simulink model "chain_CPG_2021a"  (R2021b)
settings: Solver=VariableStepAuto  StartTime=0.0  StopTime=10  RelTol=1e-3
values from neighbouring files (symbols this model uses):
  ar = 2    [Snake5animal.m]    (also in animal.m; parameters.m)
  ax = 2    [Snake5animal.m]    (also in animal.m; parameters.m)
  l = 1    [Snake5animal.m]    (also in animal.m = 0.5; parameters.m)
  N = 5    [Snake5animal.m]
  omega = ones(1,N)*0.6*pi    [Snake5animal.m]    (also in animal.m = ones(3,3)*2; parameters.m = ones(3,3)*2)
  omega1 = 0.6*pi    (= 1.88495559215)    [animal.m]    (also in parameters.m)
  omega2 = 0.6*pi    (= 1.88495559215)    [animal.m]    (also in parameters.m)
  omega3 = 0.6*pi    (= 1.88495559215)    [animal.m]    (also in parameters.m)
  phi = ones(3,3)*PHI    [animal.m]    (also in parameters.m)
  R1 = R1    [animal.m]    (also in parameters.m = 0.5708)
  R2 = R2    [animal.m]    (also in parameters.m = 0.5348)
  R3 = R3    [animal.m]    (also in parameters.m = 0.3731)
  X = zeros(1,N)    [Snake5animal.m]
  X1 = 0    [animal.m]    (also in parameters.m)
  X2 = 0    [animal.m]    (also in parameters.m)
  X3 = 0    [animal.m]    (also in parameters.m)
undefined symbols (not defined in the file or in its folder): Y, Z
libraries: sm_lib x23, nesl_utility x6
(part 1 of 2)
settings Model: Creator=xizh0002  LastModifiedBy=xizh0002

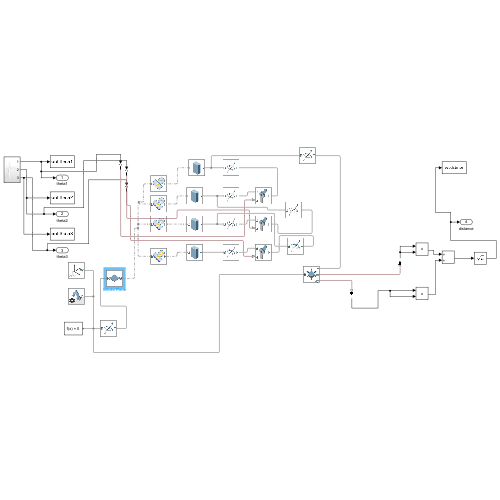
[thumbnail: Simulink's stored preview of the top-level diagram]
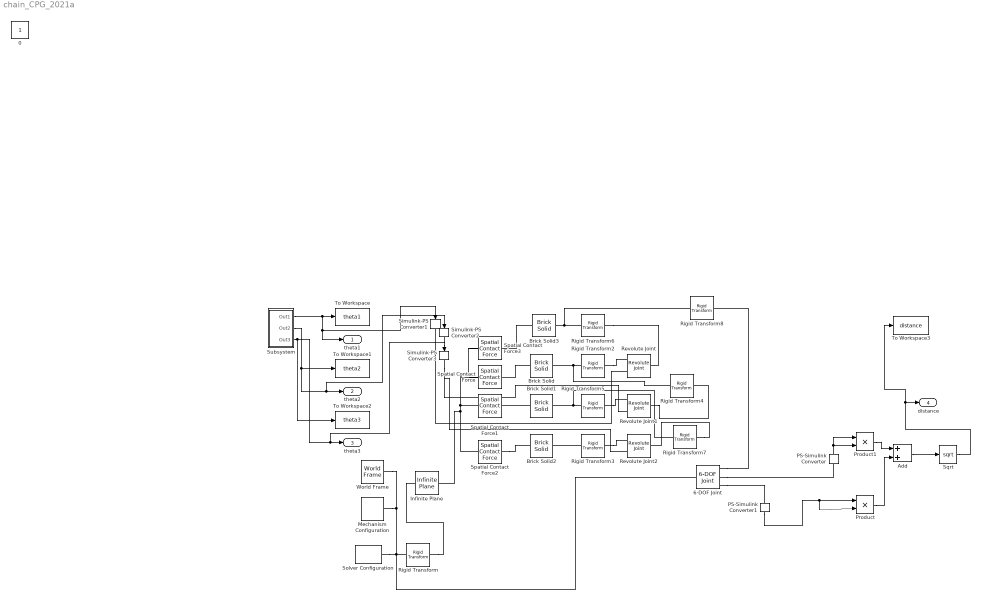
== system chain_CPG_2021a ==
  6-DOF Joint : sm_lib/Joints/6-DOF Joint  JointMode=Normal  SenseConstraintForce=off  SenseConstraintForceX=off  SenseConstraintForceY=off  SenseConstraintForceZ=off  SenseConstraintTorque=off  SenseConstraintTorqueX=off  SenseConstraintTorqueY=off  SenseConstraintTorqueZ=off  SenseTotalForce=off  SenseTotalForceX=off  SenseTotalForceY=off  SenseTotalForceZ=off  SenseTotalTorque=off  SenseTotalTorqueX=off  SenseTotalTorqueY=off  SenseTotalTorqueZ=off  CompositeWrenchDir=FollowerOnBase  CompositeWrenchFrame=BaseFrame  PxEquilibriumPosition=0  PxEquilibriumPositionUnits=m  PxSpringStiffness=0  PxSpringStiffnessUnits=N/m  PxDampingCoefficient=0  PxDampingCoefficientUnits=N/(m/s)  PxTorqueActuationMode=NoTorque  PxMotionActuationMode=ComputedMotion  PxSensePosition=on  PxSenseVelocity=off  PxSenseAcceleration=off  PxSenseTorqueForce=off  PxSenseLowerLimitTorqueForce=off  PxSenseUpperLimitTorqueForce=off  PxLowerLimitSpecify=off  PxLowerLimitBound=-1  PxLowerLimitBoundUnits=m  PxLowerLimitStiffness=1e6  PxLowerLimitStiffnessUnits=N/m  PxLowerLimitDamping=1e3  PxLowerLimitDampingUnits=N/(m/s)  PxLowerLimitTransitionRegionWidth=1e-4  PxLowerLimitTransitionRegionWidthUnits=m  PxUpperLimitSpecify=off  PxUpperLimitBound=1  PxUpperLimitBoundUnits=m  PxUpperLimitStiffness=1e6  PxUpperLimitStiffnessUnits=N/m  PxUpperLimitDamping=1e3  PxUpperLimitDampingUnits=N/(m/s)  PxUpperLimitTransitionRegionWidth=1e-4  PxUpperLimitTransitionRegionWidthUnits=m  PxPositionTargetSpecify=off  PxPositionTargetPriority=High  PxPositionTargetValue=0  PxPositionTargetValueUnits=m  PxVelocityTargetSpecify=off  PxVelocityTargetPriority=High  PxVelocityTargetValue=0  PxVelocityTargetValueUnits=m/s  PyEquilibriumPosition=0  PyEquilibriumPositionUnits=m  PySpringStiffness=0  PySpringStiffnessUnits=N/m  PyDampingCoefficient=0  PyDampingCoefficientUnits=N/(m/s)  PyTorqueActuationMode=NoTorque  PyMotionActuationMode=ComputedMotion  PySensePosition=on  PySenseVelocity=off  PySenseAcceleration=off  PySenseTorqueForce=off  PySenseLowerLimitTorqueForce=off  PySenseUpperLimitTorqueForce=off  PyLowerLimitSpecify=off  PyLowerLimitBound=-1  PyLowerLimitBoundUnits=m  PyLowerLimitStiffness=1e6  PyLowerLimitStiffnessUnits=N/m  PyLowerLimitDamping=1e3  PyLowerLimitDampingUnits=N/(m/s)  PyLowerLimitTransitionRegionWidth=1e-4  PyLowerLimitTransitionRegionWidthUnits=m  PyUpperLimitSpecify=off  PyUpperLimitBound=1  PyUpperLimitBoundUnits=m  PyUpperLimitStiffness=1e6  PyUpperLimitStiffnessUnits=N/m  PyUpperLimitDamping=1e3  PyUpperLimitDampingUnits=N/(m/s)  PyUpperLimitTransitionRegionWidth=1e-4  PyUpperLimitTransitionRegionWidthUnits=m  PyPositionTargetSpecify=off  PyPositionTargetPriority=High  PyPositionTargetValue=0  PyPositionTargetValueUnits=m  PyVelocityTargetSpecify=off  PyVelocityTargetPriority=High  PyVelocityTargetValue=0  PyVelocityTargetValueUnits=m/s  PzEquilibriumPosition=0  PzEquilibriumPositionUnits=m  PzSpringStiffness=0  PzSpringStiffnessUnits=N/m  PzDampingCoefficient=0  PzDampingCoefficientUnits=N/(m/s)  PzTorqueActuationMode=NoTorque  PzMotionActuationMode=ComputedMotion  PzSensePosition=off  PzSenseVelocity=off  PzSenseAcceleration=off  PzSenseTorqueForce=off  PzSenseLowerLimitTorqueForce=off  PzSenseUpperLimitTorqueForce=off  PzLowerLimitSpecify=off  PzLowerLimitBound=-1  PzLowerLimitBoundUnits=m  PzLowerLimitStiffness=1e6  PzLowerLimitStiffnessUnits=N/m  PzLowerLimitDamping=1e3  PzLowerLimitDampingUnits=N/(m/s)  PzLowerLimitTransitionRegionWidth=1e-4  PzLowerLimitTransitionRegionWidthUnits=m  PzUpperLimitSpecify=off  PzUpperLimitBound=1  PzUpperLimitBoundUnits=m  PzUpperLimitStiffness=1e6  PzUpperLimitStiffnessUnits=N/m  PzUpperLimitDamping=1e3  PzUpperLimitDampingUnits=N/(m/s)  PzUpperLimitTransitionRegionWidth=1e-4  PzUpperLimitTransitionRegionWidthUnits=m  PzPositionTargetSpecify=on  PzPositionTargetPriority=High  PzPositionTargetValue=l*0.7  PzPositionTargetValueUnits=m  PzVelocityTargetSpecify=off  PzVelocityTargetPriority=High  PzVelocityTargetValue=0  PzVelocityTargetValueUnits=m/s  SphDefPosRotationMethod=None  SphDefPosRotationAngleUnits=deg  SphDefPosRotationStandardAxis=+Z  SphDefPosRotationAngle=0.0  SphDefPosRotationArbitraryAxis=[0 0 1]  SphDefPosFollAlignAxisA=+X  SphDefPosBaseAlignAxisA=+Y  SphDefPosFollAlignAxisB=+Y  SphDefPosBaseAlignAxisB=+Z  SphDefPosRotationSequenceAxes=FollowerAxes  SphDefPosRotationSequence=XYX  SphDefPosRotationSequenceAngles=[0 0 0]  SphDefPosRotationSequenceAnglesUnits=deg  SphDefPosRotationMatrix=[1 0 0; 0 1 0; 0 0 1]  SphEqPosRotationMethod=None  SphEqPosRotationAngleUnits=deg  SphEqPosRotationStandardAxis=+Z  SphEqPosRotationAngle=0.0  SphEqPosRotationArbitraryAxis=[0 0 1]  SphEqPosFollAlignAxisA=+X  SphEqPosBaseAlignAxisA=+Y  SphEqPosFollAlignAxisB=+Y  SphEqPosBaseAlignAxisB=+Z  SphEqPosRotationSequenceAxes=FollowerAxes  SphEqPosRotationSequence=XYX  SphEqPosRotationSequenceAngles=[0 0 0]  SphEqPosRotationSequenceAnglesUnits=deg  SphEqPosRotationMatrix=[1 0 0; 0 1 0; 0 0 1]  SphSpringStiffness=0  SphSpringStiffnessUnits=N*m/deg  SphDampingCoefficient=0  SphDampingCoefficientUnits=N*m/(deg/s)  SphActuateTorqueX=off  SphActuateTorqueY=off  SphActuateTorqueZ=off  SphActuateTorque=off  SphTorqueActuationMode=NoTorque  SphMotionActuationMode=ComputedMotion  SphActuationFrame=BaseFrame  SphSensePosition=off  SphSenseVelocityX=off  SphSenseVelocityY=off  SphSenseVelocityZ=off  SphSenseVelocity=off  SphSenseAccelerationX=off  SphSenseAccelerationY=off  SphSenseAccelerationZ=off  SphSenseAcceleration=off  SphSenseTorqueX=off  SphSenseTorqueY=off  SphSenseTorqueZ=off  SphSenseTorqueForce=off  SphSenseLowerLimitTorqueMag=off  SphSenseUpperLimitTorqueMag=off  SphSensingFrame=BaseFrame  SphLowerLimitSpecify=off  SphLowerLimitBound=15  SphLowerLimitBoundUnits=deg  SphLowerLimitStiffness=1e4  SphLowerLimitStiffnessUnits=N*m/deg  SphLowerLimitDamping=10  SphLowerLimitDampingUnits=N*m/(deg/s)  SphLowerLimitTransitionRegionWidth=0.1  SphLowerLimitTransitionRegionWidthUnits=deg  SphUpperLimitSpecify=off  SphUpperLimitBound=45  SphUpperLimitBoundUnits=deg  SphUpperLimitStiffness=1e4  SphUpperLimitStiffnessUnits=N*m/deg  SphUpperLimitDamping=10  SphUpperLimitDampingUnits=N*m/(deg/s)  SphUpperLimitTransitionRegionWidth=0.1  SphUpperLimitTransitionRegionWidthUnits=deg  SphPositionTargetRotationMethod=None  SphPositionTargetRotationAngleUnits=deg  SphPositionTargetRotationStandardAxis=+Z  SphPositionTargetRotationAngle=0.0  SphPositionTargetRotationArbitraryAxis=[0 0 1]  SphPositionTargetFollAlignAxisA=+X  SphPositionTargetBaseAlignAxisA=+Y  SphPositionTargetFollAlignAxisB=+Y  SphPositionTargetBaseAlignAxisB=+Z  SphPositionTargetRotationSequenceAxes=FollowerAxes  SphPositionTargetRotationSequence=XYX  SphPositionTargetRotationSequenceAngles=[0 0 0]  SphPositionTargetRotationSequenceAnglesUnits=deg  SphPositionTargetRotationMatrix=[1 0 0; 0 1 0; 0 0 1]  SphPositionTargetSpecify=off  SphPositionTargetPriority=High  SphVelocityTargetValue=[0 0 0]  SphVelocityTargetValueUnits=deg/s  SphVelocityTargetSpecify=off  SphVelocityTargetPriority=High  SphVelocityTargetInFollowerFrame=on
  Add : Sum
  Brick Solid : sm_lib/Body Elements/Brick Solid  GraphicAmbientColor=[0.15 0.15 0.15 1.0]  BasedOnType=Density  BrickDimensions=[0.7 0.7 1]*l  BrickDimensionUnits=m  CenterOfMass=[0 0 0]  CenterOfMassUnits=m  GraphicDiffuseColor=[0.6 0.6 1.0]  Density=1000  DensityUnits=kg/m^3  DoExposeReferenceFrame=on  GraphicEmissiveColor=[0.0 0.0 0.0 1.0]  ExportEntireGeometry=on  SerializedFrames=<Frames/>  MarkerShape=Sphere  MarkerSize=10  GraphicType=FromGeometry  InertiaType=CalculateFromGeometry  Mass=1  MassUnits=kg  MomentsOfInertia=[1 1 1]  MomentsOfInertiaUnits=kg*m^2  GraphicOpacity=1.0  ProductsOfInertia=[0 0 0]  ProductsOfInertiaUnits=kg*m^2  GraphicShininess=75  GraphicSpecularColor=[0.5 0.5 0.5 1.0]  GraphicVisPropType=SimpleVisualProperties
  Brick Solid1 : sm_lib/Body Elements/Brick Solid  GraphicAmbientColor=[0.15 0.15 0.15 1.0]  BasedOnType=Density  BrickDimensions=[0.7 0.7 1]*l  BrickDimensionUnits=m  CenterOfMass=[0 0 0]  CenterOfMassUnits=m  GraphicDiffuseColor=[1.0 0.8 1.0]  Density=1000  DensityUnits=kg/m^3  DoExposeReferenceFrame=on  GraphicEmissiveColor=[0.0 0.0 0.0 1.0]  ExportEntireGeometry=on  SerializedFrames=<Frames/>  MarkerShape=Sphere  MarkerSize=10  GraphicType=FromGeometry  InertiaType=CalculateFromGeometry  Mass=1  MassUnits=kg  MomentsOfInertia=[1 1 1]  MomentsOfInertiaUnits=kg*m^2  GraphicOpacity=1.0  ProductsOfInertia=[0 0 0]  ProductsOfInertiaUnits=kg*m^2  GraphicShininess=75  GraphicSpecularColor=[0.5 0.5 0.5 1.0]  GraphicVisPropType=SimpleVisualProperties
  Brick Solid2 : sm_lib/Body Elements/Brick Solid  GraphicAmbientColor=[0.15 0.15 0.15 1.0]  BasedOnType=Density  BrickDimensions=[0.7 0.7 1]*l  BrickDimensionUnits=m  CenterOfMass=[0 0 0]  CenterOfMassUnits=m  GraphicDiffuseColor=[0.8 1.0 0.8]  Density=1000  DensityUnits=kg/m^3  DoExposeReferenceFrame=on  GraphicEmissiveColor=[0.0 0.0 0.0 1.0]  ExportEntireGeometry=on  SerializedFrames=<Frames/>  MarkerShape=Sphere  MarkerSize=10  GraphicType=FromGeometry  InertiaType=CalculateFromGeometry  Mass=1  MassUnits=kg  MomentsOfInertia=[1 1 1]  MomentsOfInertiaUnits=kg*m^2  GraphicOpacity=1.0  ProductsOfInertia=[0 0 0]  ProductsOfInertiaUnits=kg*m^2  GraphicShininess=75  GraphicSpecularColor=[0.5 0.5 0.5 1.0]  GraphicVisPropType=SimpleVisualProperties
  Brick Solid3 : sm_lib/Body Elements/Brick Solid  GraphicAmbientColor=[0.15 0.15 0.15 1.0]  BasedOnType=Density  BrickDimensions=[0.7 0.7 1]*l  BrickDimensionUnits=m  CenterOfMass=[0 0 0]  CenterOfMassUnits=m  GraphicDiffuseColor=[0.0 0.6 0.4]  Density=1000  DensityUnits=kg/m^3  DoExposeReferenceFrame=on  GraphicEmissiveColor=[0.0 0.0 0.0 1.0]  ExportEntireGeometry=on  SerializedFrames=<Frames/>  MarkerShape=Sphere  MarkerSize=10  GraphicType=FromGeometry  InertiaType=CalculateFromGeometry  Mass=1  MassUnits=kg  MomentsOfInertia=[1 1 1]  MomentsOfInertiaUnits=kg*m^2  GraphicOpacity=1.0  ProductsOfInertia=[0 0 0]  ProductsOfInertiaUnits=kg*m^2  GraphicShininess=75  GraphicSpecularColor=[0.5 0.5 0.5 1.0]  GraphicVisPropType=SimpleVisualProperties
  Infinite Plane : sm_lib/Curves and Surfaces/Infinite Plane  GraphicType=Rectangle  GraphicPlaneWidth=20*l  GraphicPlaneWidthUnits=m  GraphicPlaneHeight=20*l  GraphicPlaneHeightUnits=m  GraphicVisPropType=SimpleVisualProperties  GraphicDiffuseColor=[0.5 0.5 0.5]  GraphicOpacity=0.25  GraphicSpecularColor=[0.5 0.5 0.5 1.0]  GraphicAmbientColor=[0.15 0.15 0.15 1.0]  GraphicEmissiveColor=[0.0 0.0 0.0 1.0]  GraphicShininess=75
  Mechanism Configuration : sm_lib/Utilities/Mechanism Configuration  UniformGravity=Constant  GravityVector=[0 0 -9.80665]  GravityUnits=m/s^2  LinearizationDelta=0.001  JointModeTransitionNonlinearIterations=2
  PS-Simulink Converter : nesl_utility/PS-Simulink Converter  PhysicalDomain=network_engine_domain  SubClassName=ps_output  LeftPortType=input  RightPortType=output  PseudoPeriodic=off  Frequencies=[]  Unit=inherit  AffineConversion=off
      settings: SourceProductBaseCode=PW,SS
  PS-Simulink Converter1 : nesl_utility/PS-Simulink Converter  PhysicalDomain=network_engine_domain  SubClassName=ps_output  LeftPortType=input  RightPortType=output  PseudoPeriodic=off  Frequencies=[]  Unit=inherit  AffineConversion=off
      settings: SourceProductBaseCode=PW,SS
  Product : Product
  Product1 : Product
  Revolute Joint : sm_lib/Joints/Revolute Joint  JointMode=Normal  SenseConstraintForce=off  SenseConstraintForceX=off  SenseConstraintForceY=off  SenseConstraintForceZ=off  SenseConstraintTorque=off  SenseConstraintTorqueX=off  SenseConstraintTorqueY=off  SenseConstraintTorqueZ=off  SenseTotalForce=off  SenseTotalForceX=off  SenseTotalForceY=off  SenseTotalForceZ=off  SenseTotalTorque=off  SenseTotalTorqueX=off  SenseTotalTorqueY=off  SenseTotalTorqueZ=off  CompositeWrenchDir=FollowerOnBase  CompositeWrenchFrame=BaseFrame  EquilibriumPosition=0  EquilibriumPositionUnits=deg  SpringStiffness=0  SpringStiffnessUnits=N*m/deg  DampingCoefficient=0  DampingCoefficientUnits=N*m/(deg/s)  TorqueActuationMode=ComputedTorque  MotionActuationMode=InputMotion  SensePosition=off  SenseVelocity=off  SenseAcceleration=off  SenseTorqueForce=off  SenseLowerLimitTorqueForce=off  SenseUpperLimitTorqueForce=off  LowerLimitSpecify=off  LowerLimitBound=-90  LowerLimitBoundUnits=deg  LowerLimitStiffness=1e4  LowerLimitStiffnessUnits=N*m/deg  LowerLimitDamping=10  LowerLimitDampingUnits=N*m/(deg/s)  LowerLimitTransitionRegionWidth=0.1  LowerLimitTransitionRegionWidthUnits=deg  UpperLimitSpecify=off  UpperLimitBound=90  UpperLimitBoundUnits=deg  UpperLimitStiffness=1e4  UpperLimitStiffnessUnits=N*m/deg  UpperLimitDamping=10  UpperLimitDampingUnits=N*m/(deg/s)  UpperLimitTransitionRegionWidth=0.1  UpperLimitTransitionRegionWidthUnits=deg  PositionTargetSpecify=off  PositionTargetPriority=High  PositionTargetValue=0  PositionTargetValueUnits=deg  VelocityTargetSpecify=off  VelocityTargetPriority=High  VelocityTargetValue=0  VelocityTargetValueUnits=deg/s
  Revolute Joint1 : sm_lib/Joints/Revolute Joint  JointMode=Normal  SenseConstraintForce=off  SenseConstraintForceX=off  SenseConstraintForceY=off  SenseConstraintForceZ=off  SenseConstraintTorque=off  SenseConstraintTorqueX=off  SenseConstraintTorqueY=off  SenseConstraintTorqueZ=off  SenseTotalForce=off  SenseTotalForceX=off  SenseTotalForceY=off  SenseTotalForceZ=off  SenseTotalTorque=off  SenseTotalTorqueX=off  SenseTotalTorqueY=off  SenseTotalTorqueZ=off  CompositeWrenchDir=FollowerOnBase  CompositeWrenchFrame=BaseFrame  EquilibriumPosition=0  EquilibriumPositionUnits=deg  SpringStiffness=0  SpringStiffnessUnits=N*m/deg  DampingCoefficient=0  DampingCoefficientUnits=N*m/(deg/s)  TorqueActuationMode=ComputedTorque  MotionActuationMode=InputMotion  SensePosition=off  SenseVelocity=off  SenseAcceleration=off  SenseTorqueForce=off  SenseLowerLimitTorqueForce=off  SenseUpperLimitTorqueForce=off  LowerLimitSpecify=off  LowerLimitBound=-90  LowerLimitBoundUnits=deg  LowerLimitStiffness=1e4  LowerLimitStiffnessUnits=N*m/deg  LowerLimitDamping=10  LowerLimitDampingUnits=N*m/(deg/s)  LowerLimitTransitionRegionWidth=0.1  LowerLimitTransitionRegionWidthUnits=deg  UpperLimitSpecify=off  UpperLimitBound=90  UpperLimitBoundUnits=deg  UpperLimitStiffness=1e4  UpperLimitStiffnessUnits=N*m/deg  UpperLimitDamping=10  UpperLimitDampingUnits=N*m/(deg/s)  UpperLimitTransitionRegionWidth=0.1  UpperLimitTransitionRegionWidthUnits=deg  PositionTargetSpecify=off  PositionTargetPriority=High  PositionTargetValue=0  PositionTargetValueUnits=deg  VelocityTargetSpecify=off  VelocityTargetPriority=High  VelocityTargetValue=0  VelocityTargetValueUnits=deg/s
  Revolute Joint2 : sm_lib/Joints/Revolute Joint  JointMode=Normal  SenseConstraintForce=off  SenseConstraintForceX=off  SenseConstraintForceY=off  SenseConstraintForceZ=off  SenseConstraintTorque=off  SenseConstraintTorqueX=off  SenseConstraintTorqueY=off  SenseConstraintTorqueZ=off  SenseTotalForce=off  SenseTotalForceX=off  SenseTotalForceY=off  SenseTotalForceZ=off  SenseTotalTorque=off  SenseTotalTorqueX=off  SenseTotalTorqueY=off  SenseTotalTorqueZ=off  CompositeWrenchDir=FollowerOnBase  CompositeWrenchFrame=BaseFrame  EquilibriumPosition=0  EquilibriumPositionUnits=deg  SpringStiffness=0  SpringStiffnessUnits=N*m/deg  DampingCoefficient=0  DampingCoefficientUnits=N*m/(deg/s)  TorqueActuationMode=ComputedTorque  MotionActuationMode=InputMotion  SensePosition=off  SenseVelocity=off  SenseAcceleration=off  SenseTorqueForce=off  SenseLowerLimitTorqueForce=off  SenseUpperLimitTorqueForce=off  LowerLimitSpecify=off  LowerLimitBound=-90  LowerLimitBoundUnits=deg  LowerLimitStiffness=1e4  LowerLimitStiffnessUnits=N*m/deg  LowerLimitDamping=10  LowerLimitDampingUnits=N*m/(deg/s)  LowerLimitTransitionRegionWidth=0.1  LowerLimitTransitionRegionWidthUnits=deg  UpperLimitSpecify=off  UpperLimitBound=90  UpperLimitBoundUnits=deg  UpperLimitStiffness=1e4  UpperLimitStiffnessUnits=N*m/deg  UpperLimitDamping=10  UpperLimitDampingUnits=N*m/(deg/s)  UpperLimitTransitionRegionWidth=0.1  UpperLimitTransitionRegionWidthUnits=deg  PositionTargetSpecify=off  PositionTargetPriority=High  PositionTargetValue=0  PositionTargetValueUnits=deg  VelocityTargetSpecify=off  VelocityTargetPriority=High  VelocityTargetValue=0  VelocityTargetValueUnits=deg/s
  Rigid Transform : sm_lib/Frames and Transforms/Rigid Transform  TranslationMethod=StandardAxis  TranslationStandardOffset=0  TranslationLengthUnit=m  TranslationStandardAxis=-Z  TranslationCartesianOffset=[0 0 0]  TranslationROffset=0  TranslationROffsetUnits=m  TranslationZOffset=0  TranslationZOffsetUnits=m  TranslationThetaOffset=0  TranslationThetaOffsetUnits=deg  RotationMethod=StandardAxis  RotationAngleUnits=deg  RotationStandardAxis=-X  RotationAngle=0  RotationArbitraryAxis=[0 0 1]  FollAlignAxisA=+X  BaseAlignAxisA=+Y  FollAlignAxisB=+Y  BaseAlignAxisB=+Z  RotationSequenceAxes=FollowerAxes  RotationSequence=XYX  RotationSequenceAngles=[0 0 0]  RotationSequenceAnglesUnits=deg  RotationMatrix=[1 0 0; 0 1 0; 0 0 1]
  Rigid Transform2 : sm_lib/Frames and Transforms/Rigid Transform  TranslationMethod=StandardAxis  TranslationStandardOffset=0.5*l  TranslationLengthUnit=m  TranslationStandardAxis=+Z  TranslationCartesianOffset=[0 0 0]  TranslationROffset=0  TranslationROffsetUnits=m  TranslationZOffset=0  TranslationZOffsetUnits=m  TranslationThetaOffset=0  TranslationThetaOffsetUnits=deg  RotationMethod=StandardAxis  RotationAngleUnits=deg  RotationStandardAxis=+X  RotationAngle=92  RotationArbitraryAxis=[0 1 0]  FollAlignAxisA=+X  BaseAlignAxisA=+Y  FollAlignAxisB=+Y  BaseAlignAxisB=+Z  RotationSequenceAxes=FollowerAxes  RotationSequence=XYX  RotationSequenceAngles=[90 90 0]  RotationSequenceAnglesUnits=deg  RotationMatrix=[1 0 0; 0 1 0; 0 0 1]
  Rigid Transform3 : sm_lib/Frames and Transforms/Rigid Transform  TranslationMethod=StandardAxis  TranslationStandardOffset=0.5*l  TranslationLengthUnit=m  TranslationStandardAxis=+Z  TranslationCartesianOffset=[0 0 0]  TranslationROffset=0  TranslationROffsetUnits=m  TranslationZOffset=0  TranslationZOffsetUnits=m  TranslationThetaOffset=0  TranslationThetaOffsetUnits=deg  RotationMethod=StandardAxis  RotationAngleUnits=deg  RotationStandardAxis=+X  RotationAngle=92  RotationArbitraryAxis=[0 0 1]  FollAlignAxisA=+X  BaseAlignAxisA=+Y  FollAlignAxisB=+Y  BaseAlignAxisB=+Z  RotationSequenceAxes=FollowerAxes  RotationSequence=XYX  RotationSequenceAngles=[0 0 0]  RotationSequenceAnglesUnits=deg  RotationMatrix=[1 0 0; 0 1 0; 0 0 1]
  Rigid Transform4 : sm_lib/Frames and Transforms/Rigid Transform  TranslationMethod=StandardAxis  TranslationStandardOffset=0.5*l  TranslationLengthUnit=m  TranslationStandardAxis=-Z  TranslationCartesianOffset=[0 0 0]  TranslationROffset=0  TranslationROffsetUnits=m  TranslationZOffset=0  TranslationZOffsetUnits=m  TranslationThetaOffset=0  TranslationThetaOffsetUnits=deg  RotationMethod=StandardAxis  RotationAngleUnits=deg  RotationStandardAxis=+X  RotationAngle=88  RotationArbitraryAxis=[0 0 1]  FollAlignAxisA=+X  BaseAlignAxisA=+Y  FollAlignAxisB=+Y  BaseAlignAxisB=+Z  RotationSequenceAxes=FollowerAxes  RotationSequence=XYX  RotationSequenceAngles=[0 0 0]  RotationSequenceAnglesUnits=deg  RotationMatrix=[1 0 0; 0 1 0; 0 0 1]
  Rigid Transform5 : sm_lib/Frames and Transforms/Rigid Transform  TranslationMethod=StandardAxis  TranslationStandardOffset=0.5*l  TranslationLengthUnit=m  TranslationStandardAxis=+Z  TranslationCartesianOffset=[0 0 0]  TranslationROffset=0  TranslationROffsetUnits=m  TranslationZOffset=0  TranslationZOffsetUnits=m  TranslationThetaOffset=0  TranslationThetaOffsetUnits=deg  RotationMethod=StandardAxis  RotationAngleUnits=deg  RotationStandardAxis=+X  RotationAngle=88  RotationArbitraryAxis=[0 0 1]  FollAlignAxisA=+X  BaseAlignAxisA=+Y  FollAlignAxisB=+Y  BaseAlignAxisB=+Z  RotationSequenceAxes=FollowerAxes  RotationSequence=XYX  RotationSequenceAngles=[0 0 0]  RotationSequenceAnglesUnits=deg  RotationMatrix=[1 0 0; 0 1 0; 0 0 1]
  Rigid Transform6 : sm_lib/Frames and Transforms/Rigid Transform  TranslationMethod=StandardAxis  TranslationStandardOffset=0.5*l  TranslationLengthUnit=m  TranslationStandardAxis=-Z  TranslationCartesianOffset=[0 0 0]  TranslationROffset=0  TranslationROffsetUnits=m  TranslationZOffset=0  TranslationZOffsetUnits=m  TranslationThetaOffset=0  TranslationThetaOffsetUnits=deg  RotationMethod=StandardAxis  RotationAngleUnits=deg  RotationStandardAxis=+X  RotationAngle=92  RotationArbitraryAxis=[0 0 1]  FollAlignAxisA=+X  BaseAlignAxisA=+Y  FollAlignAxisB=+Y  BaseAlignAxisB=+Z  RotationSequenceAxes=FollowerAxes  RotationSequence=XYX  RotationSequenceAngles=[0 0 0]  RotationSequenceAnglesUnits=deg  RotationMatrix=[1 0 0; 0 1 0; 0 0 1]
  Rigid Transform7 : sm_lib/Frames and Transforms/Rigid Transform  TranslationMethod=StandardAxis  TranslationStandardOffset=0.5*l  TranslationLengthUnit=m  TranslationStandardAxis=-Z  TranslationCartesianOffset=[0 0 0]  TranslationROffset=0  TranslationROffsetUnits=m  TranslationZOffset=0  TranslationZOffsetUnits=m  TranslationThetaOffset=0  TranslationThetaOffsetUnits=deg  RotationMethod=StandardAxis  RotationAngleUnits=deg  RotationStandardAxis=+X  RotationAngle=92  RotationArbitraryAxis=[0 0 1]  FollAlignAxisA=+X  BaseAlignAxisA=+Y  FollAlignAxisB=+Y  BaseAlignAxisB=+Z  RotationSequenceAxes=FollowerAxes  RotationSequence=XYX  RotationSequenceAngles=[0 0 0]  RotationSequenceAnglesUnits=deg  RotationMatrix=[1 0 0; 0 1 0; 0 0 1]
  Rigid Transform8 : sm_lib/Frames and Transforms/Rigid Transform  TranslationMethod=StandardAxis  TranslationStandardOffset=0  TranslationLengthUnit=m  TranslationStandardAxis=+Z  TranslationCartesianOffset=[0 0 0]  TranslationROffset=0  TranslationROffsetUnits=m  TranslationZOffset=0  TranslationZOffsetUnits=m  TranslationThetaOffset=0  TranslationThetaOffsetUnits=deg  RotationMethod=StandardAxis  RotationAngleUnits=deg  RotationStandardAxis=-Y  RotationAngle=90  RotationArbitraryAxis=[0 1 0]  FollAlignAxisA=+X  BaseAlignAxisA=+Y  FollAlignAxisB=+Y  BaseAlignAxisB=+Z  RotationSequenceAxes=FollowerAxes  RotationSequence=XYX  RotationSequenceAngles=[90 90 0]  RotationSequenceAnglesUnits=deg  RotationMatrix=[1 0 0; 0 1 0; 0 0 1]
  Simulink-PS Converter1 : nesl_utility/Simulink-PS Converter  PhysicalDomain=network_engine_domain  SubClassName=ps_input  LeftPortType=input  RightPortType=output  PseudoPeriodic=off  Frequencies=[]  NoiseDistribution=none  NoiseParameters=[]  Unit=1  AffineConversion=off  FilteringAndDerivatives=filter  SimscapeFilterOrder=2  InputFilterTimeConstant=0.001  UdotUserProvided=0
      settings: SourceProductBaseCode=PW,SS
  Simulink-PS Converter2 : nesl_utility/Simulink-PS Converter  PhysicalDomain=network_engine_domain  SubClassName=ps_input  LeftPortType=input  RightPortType=output  PseudoPeriodic=off  Frequencies=[]  NoiseDistribution=none  NoiseParameters=[]  Unit=1  AffineConversion=off  FilteringAndDerivatives=filter  SimscapeFilterOrder=2  InputFilterTimeConstant=0.001  UdotUserProvided=0
      settings: SourceProductBaseCode=PW,SS
  Simulink-PS Converter3 : nesl_utility/Simulink-PS Converter  PhysicalDomain=network_engine_domain  SubClassName=ps_input  LeftPortType=input  RightPortType=output  PseudoPeriodic=off  Frequencies=[]  NoiseDistribution=none  NoiseParameters=[]  Unit=1  AffineConversion=off  FilteringAndDerivatives=filter  SimscapeFilterOrder=2  InputFilterTimeConstant=0.001  UdotUserProvided=0
      settings: SourceProductBaseCode=PW,SS
  Solver Configuration : nesl_utility/Solver Configuration  PhysicalDomain=network_engine_domain  SubClassName=solver  LeftPortType=input  RightPortType=generic  Tones=[]  Harmonics=[]  SimulateNoise=off  Profile=off  UseLocalSampling=off  EnableSwitchedLinearOptims=on  FrequencyDomain=off  UseCCode=off  RelTol=0.001  AbsTol=0.001  MinStep=1e-09  ToWorkspace=off  RevertToSquareIcSolve=off  NumHomotopyIterations=100  PhasorMode=off  PhasorModeNumHarmonics=1  DoDC=off  ResidualTolerance=1e-09  UseLocalSolver=off  LocalSolverChoice=NE_BACKWARD_EULER_ADVANCER  LocalSolverSampleTime=0.001  DoFixedCost=off  MaxNonlinIter=3  MaxModeIter=2  ComputeImpulses=off  ImpulseIterations=2  LinearAlgebra=auto  EquationFormulation=NE_TIME_EF  DelaysMemoryBudget=1024  AutomaticFiltering=on  FilteringTimeConstant=0.001  PartitionStorageMethod=AS_NEEDED  PartitionMemoryBudget=1024  PartitionMethod=ROBUST
      settings: SourceProductBaseCode=PW,SS
  Spatial Contact Force{,1..3} (4 alike) : sm_lib/Forces and Torques/Spatial Contact Force  CoefficientOfDynamicFriction=0.3  CoefficientOfStaticFriction=0.5  SenseContactBaseRotation=off  SenseContactBaseTranslation=off  NormalDamping=1e3  NormalDampingUnits=N/(m/s)  SenseContactFollowerRotation=off  SenseContactFollowerTranslation=off  SenseContactSignal=off  NormalStiffness=1e5  NormalStiffnessUnits=N/m  FrictionalCriticalVelocity=1e-3  FrictionalCriticalVelocityUnits=m/s  ZeroCrossDetectContactStartAndEnd=off  FrictionType=SmoothStickSlip  SenseFrictionalForceMagnitude=off  SenseNormalForceMagnitude=off  NormalForceType=SmoothSpringDamper  SenseNormalVelocity=off  SenseSeparationDistance=off  SenseTangentialVelocity=off  SenseTangentialVelocityMagnitude=off  NormalTransitionRegionWidth=1e-4  NormalTransitionRegionWidthUnits=m
  Sqrt : Sqrt  SaturateOnIntegerOverflow=on
  Subsystem : Subsystem
  To Workspace : ToWorkspace  VariableName=theta1  SaveFormat=Timeseries  SampleTime=-1
  To Workspace1 : ToWorkspace  VariableName=theta2  SaveFormat=Timeseries  SampleTime=-1
  To Workspace2 : ToWorkspace  VariableName=theta3  SaveFormat=Timeseries  SampleTime=-1
  To Workspace3 : ToWorkspace  VariableName=distance  SaveFormat=Timeseries  SampleTime=-1
  World Frame : sm_lib/Frames and Transforms/World Frame
  theta1 : Outport
  theta2 : Outport  Port=2
  theta3 : Outport  Port=3
  distance : Outport  Port=4
  "0 " : Constant  IOType=siggen
  wires:
  Subsystem/1(Out1) -> To Workspace/1, Simulink-PS Converter1/1, theta1/1
  Subsystem/2(Out2) -> To Workspace1/1, Simulink-PS Converter2/1, theta2/1
  Subsystem/3(Out3) -> To Workspace2/1, Simulink-PS Converter3/1, theta3/1
  PS-Simulink Converter1/1 -> Product/2, Product/1
  PS-Simulink Converter/1 -> Product1/2, Product1/1
  Product1/1 -> Add/1
  Product/1 -> Add/2
  Add/1 -> Sqrt/1
  Sqrt/1 -> To Workspace3/1, distance/1
  connections:
  Spatial Contact Force/LConn1 -- Spatial Contact Force3/LConn1 -- Spatial Contact Force2/LConn1 -- Infinite Plane/RConn1 -- Spatial Contact Force1/LConn1
  Brick Solid/LConn1 -- Spatial Contact Force/RConn1
  Brick Solid1/LConn1 -- Spatial Contact Force1/RConn1
  Spatial Contact Force2/RConn1 -- Brick Solid2/LConn1
  Rigid Transform/RConn1 -- Infinite Plane/LConn1
  Rigid Transform5/RConn1 -- Revolute Joint1/LConn1
  Rigid Transform3/RConn1 -- Revolute Joint2/LConn1
  Rigid Transform2/LConn1 -- Rigid Transform4/LConn1 -- Brick Solid/RConn1
  Rigid Transform2/RConn1 -- Revolute Joint/LConn1
  Rigid Transform5/LConn1 -- Rigid Transform7/LConn1 -- Brick Solid1/RConn1
  Rigid Transform3/LConn1 -- Brick Solid2/RConn1
  Brick Solid3/LConn1 -- Spatial Contact Force3/RConn1
  Revolute Joint/LConn2 -- Simulink-PS Converter1/RConn1
  Simulink-PS Converter2/RConn1 -- Revolute Joint1/LConn2
  Simulink-PS Converter3/RConn1 -- Revolute Joint2/LConn2
  6-DOF Joint/RConn2 -- PS-Simulink Converter/LConn1
  6-DOF Joint/RConn3 -- PS-Simulink Converter1/LConn1
  Rigid Transform7/RConn1 -- Revolute Joint2/RConn1
  Revolute Joint1/RConn1 -- Rigid Transform4/RConn1
  Rigid Transform6/RConn1 -- Revolute Joint/RConn1
  Rigid Transform6/LConn1 -- Rigid Transform8/LConn1 -- Brick Solid3/RConn1
  6-DOF Joint/RConn1 -- Rigid Transform8/RConn1
  World Frame/RConn1 -- 6-DOF Joint/LConn1 -- Rigid Transform/LConn1 -- Solver Configuration/RConn1 -- Mechanism Configuration/RConn1

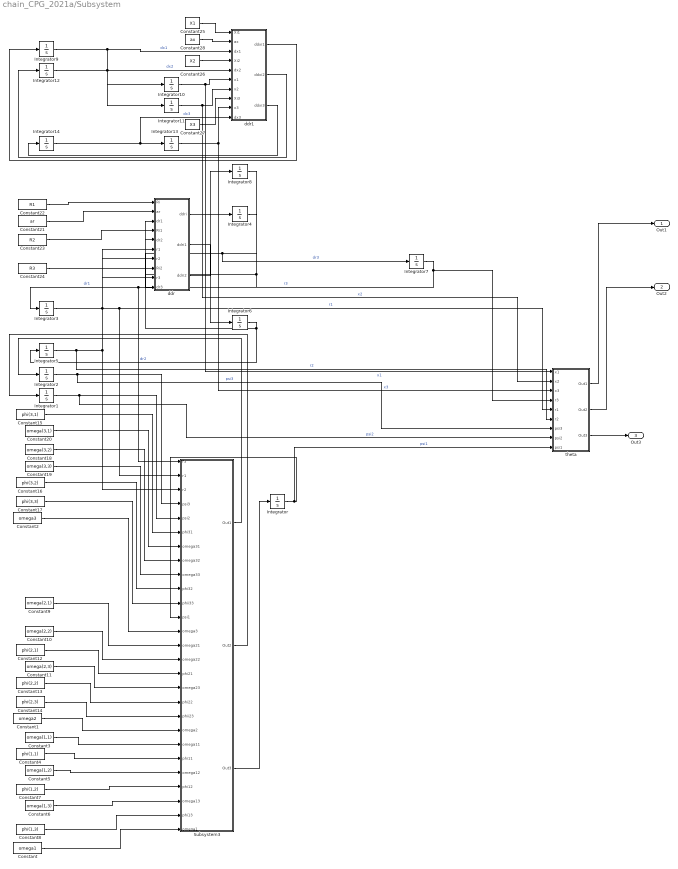
== system chain_CPG_2021a/Subsystem ==
  Constant : Constant  Value=omega1
  Constant1 : Constant  Value=omega2
  Constant10 : Constant  Value=omega(2,2)
  Constant11 : Constant  Value=omega(2,3)
  Constant12 : Constant  Value=phi(2,1)
  Constant13 : Constant  Value=phi(2,2)
  Constant14 : Constant  Value=phi(2,3)
  Constant15 : Constant  Value=phi(3,1)
  Constant16 : Constant  Value=phi(3,2)
  Constant17 : Constant  Value=phi(3,3)
  Constant18 : Constant  Value=omega(3,2)
  Constant19 : Constant  Value=omega(3,3)
  Constant2 : Constant  Value=omega3
  Constant20 : Constant  Value=omega(3,1)
  Constant21 : Constant  Value=ar
  Constant22 : Constant  Value=R1
  Constant23 : Constant  Value=R2
  Constant24 : Constant  Value=R3
  Constant25 : Constant  Value=X1
  Constant26 : Constant  Value=X2
  Constant27 : Constant  Value=X3
  Constant28 : Constant  Value=ax
  Constant3 : Constant  Value=omega(1,1)
  Constant4 : Constant  Value=phi(1,1)
  Constant5 : Constant  Value=omega(1,2)
  Constant6 : Constant  Value=omega(1,3)
  Constant7 : Constant  Value=phi(1,2)
  Constant8 : Constant  Value=phi(1,3)
  Constant9 : Constant  Value=omega(2,1)
  Integrator{,1..14} (15 alike) : Integrator
  Subsystem3 : Subsystem
  ddr : Subsystem
  ddr1 : Subsystem
  theta : Subsystem
  Out1 : Outport
  Out2 : Outport  Port=2
  Out3 : Outport  Port=3
  wires:
  Subsystem3/3(Out3) -> Integrator/1
  Integrator11/1 -> theta/2(x2), ddr1/7(x2)  "x2"
  Constant24/1 -> ddr/8(Ri2)
  Constant28/1 -> ddr1/2(ax)
  Integrator12/1 -> Integrator11/1, ddr1/5(dx2)  "dx2"
  Integrator1/1 -> theta/8(psi2), Subsystem3/5(psi2)  "psi2"
  theta/2(Out2) -> Out2/1
  Integrator9/1 -> ddr1/3(dx1), Integrator10/1  "dx1"
  Integrator14/1 -> Integrator13/1, ddr1/10(dx3)  "dx3"
  ddr1/1(ddxi1) -> Integrator9/1
  Constant27/1 -> ddr1/8(Xi3)
  Subsystem3/2(Out2) -> Integrator1/1
  Integrator13/1 -> ddr1/9(x3), theta/3(x3)  "x3"
  Constant14/1 -> Subsystem3/19(phii23)
  ddr1/2(ddxi2) -> Integrator12/1
  Integrator6/1 -> ddr/5(dr2), Integrator5/1  "dr2"
  Integrator/1 -> theta/9(psi1), Subsystem3/12(psi1)  "psi1"
  Integrator10/1 -> theta/1(x1), ddr1/6(x1)  "x1"
  ddr1/3(ddxi3) -> Integrator14/1
  ddr/3(ddri2) -> Integrator8/1
  Integrator3/1 -> theta/5(r1), Subsystem3/2(r1), ddr/6(r1)  "r1"
  Constant10/1 -> Subsystem3/15(omega22)
  Integrator4/1 -> ddr/3(dr1), Integrator3/1  "dr1"
  Constant17/1 -> Subsystem3/11(phii33)
  Integrator5/1 -> theta/6(r2), Subsystem3/3(r2), ddr/7(r2)  "r2"
  Constant16/1 -> Subsystem3/10(phi32)
  Constant18/1 -> Subsystem3/8(omega32)
  Integrator8/1 -> ddr/10(dr3), Integrator7/1  "dr3"
  Integrator2/1 -> theta/7(psi3), Subsystem3/4(psi3)  "psi3"
  Constant22/1 -> ddr/1(Ri)
  Constant7/1 -> Subsystem3/24(phi12)
  Constant11/1 -> Subsystem3/17(omega23)
  Constant2/1 -> Subsystem3/13(omega3)
  Constant4/1 -> Subsystem3/22(phi11)
  Constant21/1 -> ddr/2(ar)
  Integrator7/1 -> theta/4(r3), ddr/9(r3), Subsystem3/1(r3)  "r3"
  Constant19/1 -> Subsystem3/9(omega33)
  Constant8/1 -> Subsystem3/26(phi13)
  Constant13/1 -> Subsystem3/18(phi22)
  ddr/2(ddri1) -> Integrator6/1
  Constant15/1 -> Subsystem3/6(phi31)
  Constant20/1 -> Subsystem3/7(omega31)
  theta/3(Out3) -> Out3/1
  ddr/1(ddri) -> Integrator4/1
  Constant9/1 -> Subsystem3/14(omega21)
  Constant6/1 -> Subsystem3/25(omega13)
  Constant23/1 -> ddr/4(Ri1)
  Constant3/1 -> Subsystem3/21(omega11)
  Constant12/1 -> Subsystem3/16(phi21)
  Constant/1 -> Subsystem3/27(omega1)
  Constant1/1 -> Subsystem3/20(omega2)
  Constant26/1 -> ddr1/4(Xi2)
  Constant25/1 -> ddr1/1(Xi1)
  Constant5/1 -> Subsystem3/23(omega12)
  Subsystem3/1(Out1) -> Integrator2/1
  theta/1(Out1) -> Out1/1

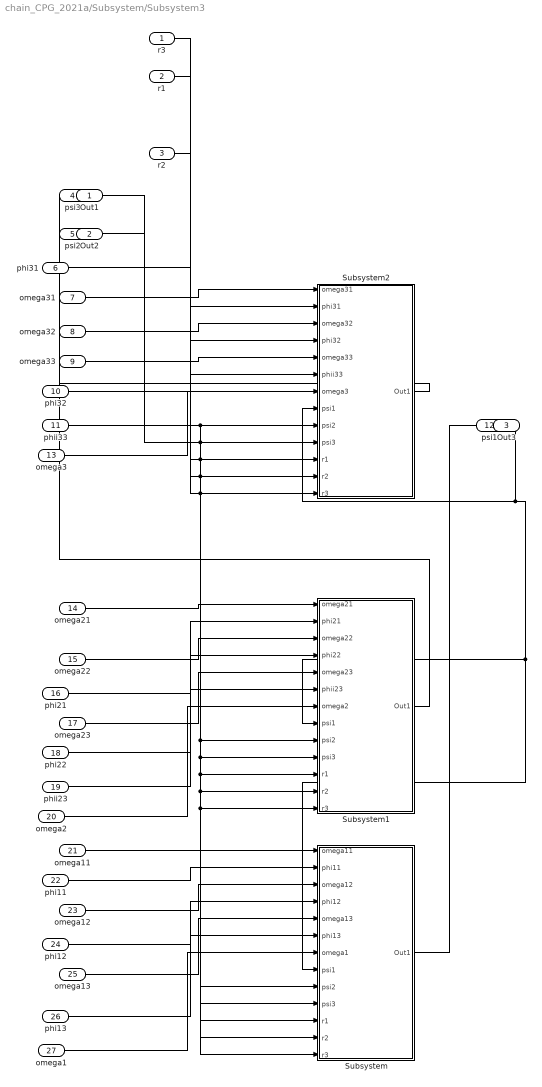
== system chain_CPG_2021a/Subsystem/Subsystem3 ==
  r3 : Inport
  r1 : Inport  Port=2
  r2 : Inport  Port=3
  psi3 : Inport  Port=4
  psi2 : Inport  Port=5
  phi31 : Inport  Port=6
  omega31 : Inport  Port=7
  omega32 : Inport  Port=8
  omega33 : Inport  Port=9
  phi32 : Inport  Port=10
  phii33 : Inport  Port=11
  psi1 : Inport  Port=12
  omega3 : Inport  Port=13
  omega21 : Inport  Port=14
  omega22 : Inport  Port=15
  phi21 : Inport  Port=16
  omega23 : Inport  Port=17
  phi22 : Inport  Port=18
  phii23 : Inport  Port=19
  omega2 : Inport  Port=20
  omega11 : Inport  Port=21
  phi11 : Inport  Port=22
  omega12 : Inport  Port=23
  phi12 : Inport  Port=24
  omega13 : Inport  Port=25
  phi13 : Inport  Port=26
  omega1 : Inport  Port=27
  Subsystem : Subsystem
  Subsystem1 : Subsystem
  Subsystem2 : Subsystem
  Out1 : Outport
  Out2 : Outport  Port=2
  Out3 : Outport  Port=3
  wires:
  omega21/1 -> Subsystem1/1(omega21)
  r2/1 -> Subsystem1/12(r2), Subsystem/12(r2), Subsystem2/12(r2)
  psi3/1 -> Subsystem1/10(psi3), Subsystem/10(psi3), Subsystem2/10(psi3)
  phi12/1 -> Subsystem/4(phi12)
  r3/1 -> Subsystem/13(r3), Subsystem1/13(r3), Subsystem2/13(r3)
  psi1/1 -> Subsystem/8(psi1), Subsystem1/8(psi1), Subsystem2/8(psi1)
  Subsystem2/1(Out1) -> Out1/1
  omega12/1 -> Subsystem/3(omega12)
  Subsystem1/1(Out1) -> Out2/1
  phi32/1 -> Subsystem2/4(phi32)
  phi22/1 -> Subsystem1/4(phi22)
  omega11/1 -> Subsystem/1(omega11)
  psi2/1 -> Subsystem/9(psi2), Subsystem1/9(psi2), Subsystem2/9(psi2)
  omega22/1 -> Subsystem1/3(omega22)
  r1/1 -> Subsystem1/11(r1), Subsystem/11(r1), Subsystem2/11(r1)
  omega13/1 -> Subsystem/5(omega13)
  omega2/1 -> Subsystem1/7(omega2)
  Subsystem/1(Out1) -> Out3/1
  omega3/1 -> Subsystem2/7(omega3)
  omega33/1 -> Subsystem2/5(omega33)
  phi13/1 -> Subsystem/6(phi13)
  phii33/1 -> Subsystem2/6(phii33)
  phi21/1 -> Subsystem1/2(phi21)
  omega32/1 -> Subsystem2/3(omega32)
  phi31/1 -> Subsystem2/2(phi31)
  phii23/1 -> Subsystem1/6(phii23)
  omega31/1 -> Subsystem2/1(omega31)
  omega1/1 -> Subsystem/7(omega1)
  omega23/1 -> Subsystem1/5(omega23)
  phi11/1 -> Subsystem/2(phi11)

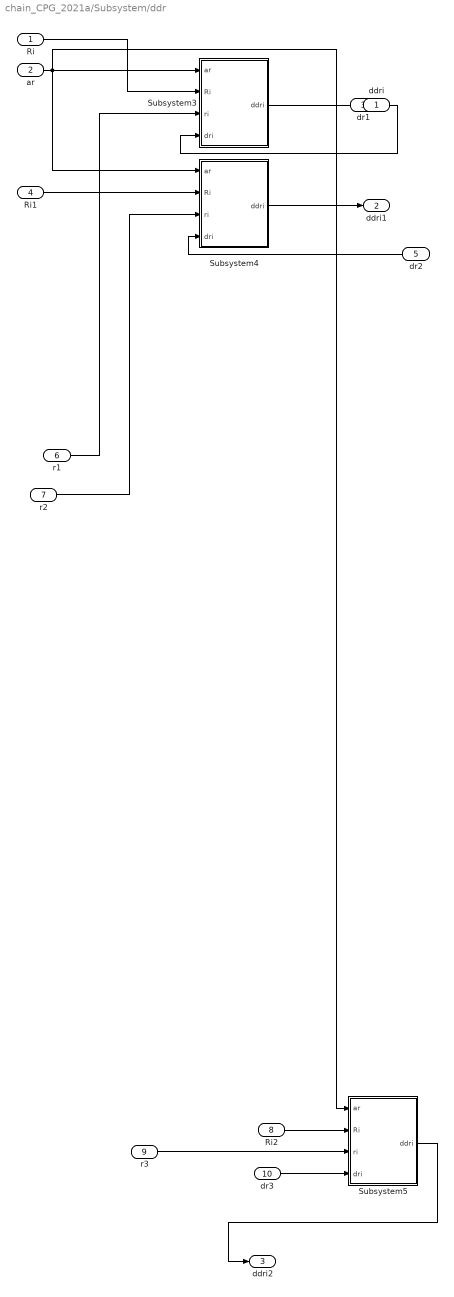
== system chain_CPG_2021a/Subsystem/ddr ==
  Ri : Inport
  ar : Inport  Port=2
  dr1 : Inport  Port=3
  Ri1 : Inport  Port=4
  dr2 : Inport  Port=5
  r1 : Inport  Port=6
  r2 : Inport  Port=7
  Ri2 : Inport  Port=8
  r3 : Inport  Port=9
  dr3 : Inport  Port=10
  Subsystem3 : Subsystem
  Subsystem4 : Subsystem
  Subsystem5 : Subsystem
  ddri : Outport
  ddri1 : Outport  Port=2
  ddri2 : Outport  Port=3
  wires:
  r1/1 -> Subsystem3/3(ri)
  Subsystem4/1(ddri) -> ddri1/1
  r3/1 -> Subsystem5/3(ri)
  ar/1 -> Subsystem4/1(ar), Subsystem5/1(ar), Subsystem3/1(ar)
  dr3/1 -> Subsystem5/4(dri)
  r2/1 -> Subsystem4/3(ri)
  Subsystem3/1(ddri) -> ddri/1
  dr1/1 -> Subsystem3/4(dri)
  Subsystem5/1(ddri) -> ddri2/1
  dr2/1 -> Subsystem4/4(dri)
  Ri1/1 -> Subsystem4/2(Ri)
  Ri2/1 -> Subsystem5/2(Ri)
  Ri/1 -> Subsystem3/2(Ri)

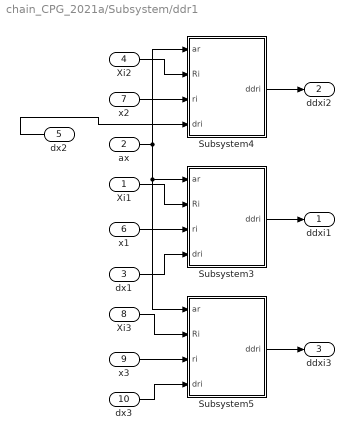
== system chain_CPG_2021a/Subsystem/ddr1 ==
  Xi1 : Inport
  ax : Inport  Port=2
  dx1 : Inport  Port=3
  Xi2 : Inport  Port=4
  dx2 : Inport  Port=5
  x1 : Inport  Port=6
  x2 : Inport  Port=7
  Xi3 : Inport  Port=8
  x3 : Inport  Port=9
  dx3 : Inport  Port=10
  Subsystem3 : Subsystem
  Subsystem4 : Subsystem
  Subsystem5 : Subsystem
  ddxi1 : Outport
  ddxi2 : Outport  Port=2
  ddxi3 : Outport  Port=3
  wires:
  Subsystem3/1(ddri) -> ddxi1/1
  Subsystem5/1(ddri) -> ddxi3/1
  Xi2/1 -> Subsystem4/2(Ri)
  Xi1/1 -> Subsystem3/2(Ri)
  x2/1 -> Subsystem4/3(ri)
  dx1/1 -> Subsystem3/4(dri)
  dx2/1 -> Subsystem4/4(dri)
  Xi3/1 -> Subsystem5/2(Ri)
  dx3/1 -> Subsystem5/4(dri)
  x3/1 -> Subsystem5/3(ri)
  Subsystem4/1(ddri) -> ddxi2/1
  x1/1 -> Subsystem3/3(ri)
  ax/1 -> Subsystem5/1(ar), Subsystem3/1(ar), Subsystem4/1(ar)

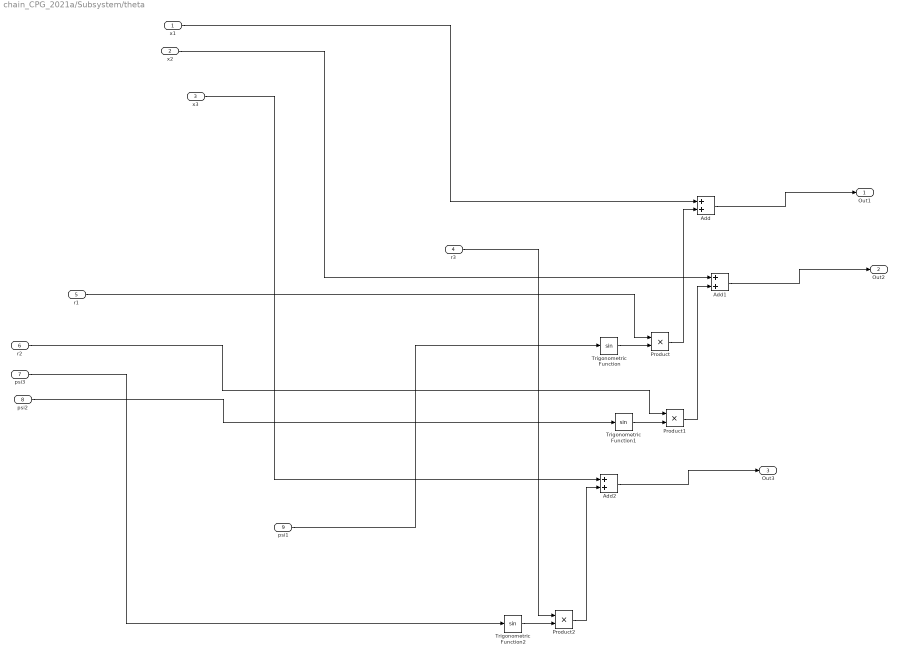
== system chain_CPG_2021a/Subsystem/theta ==
  x1 : Inport
  x2 : Inport  Port=2
  x3 : Inport  Port=3
  r3 : Inport  Port=4
  r1 : Inport  Port=5
  r2 : Inport  Port=6
  psi3 : Inport  Port=7
  psi2 : Inport  Port=8
  psi1 : Inport  Port=9
  Add : Sum
  Add1 : Sum
  Add2 : Sum
  Product : Product
  Product1 : Product
  Product2 : Product
  Trigonometric Function : Trigonometry
  Trigonometric Function1 : Trigonometry
  Trigonometric Function2 : Trigonometry
  Out1 : Outport
  Out2 : Outport  Port=2
  Out3 : Outport  Port=3
  wires:
  Product2/1 -> Add2/2
  Product/1 -> Add/2
  Trigonometric Function2/1 -> Product2/2
  Trigonometric Function1/1 -> Product1/2
  Add1/1 -> Out2/1
  psi3/1 -> Trigonometric Function2/1
  Product1/1 -> Add1/2
  psi1/1 -> Trigonometric Function/1
  Trigonometric Function/1 -> Product/2
  r3/1 -> Product2/1
  Add/1 -> Out1/1
  r2/1 -> Product1/1
  x1/1 -> Add/1
  psi2/1 -> Trigonometric Function1/1
  r1/1 -> Product/1
  x3/1 -> Add2/1
  Add2/1 -> Out3/1
  x2/1 -> Add1/1

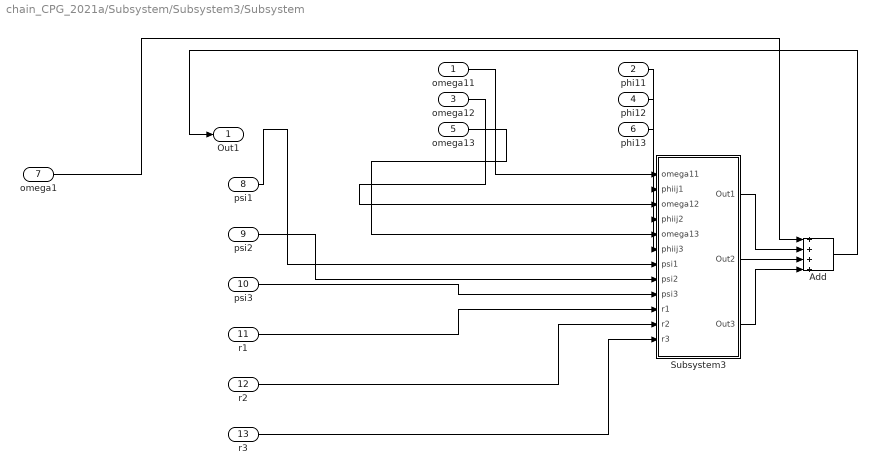
== system chain_CPG_2021a/Subsystem/Subsystem3/Subsystem ==
  omega11 : Inport
  phi11 : Inport  Port=2
  omega12 : Inport  Port=3
  phi12 : Inport  Port=4
  omega13 : Inport  Port=5
  phi13 : Inport  Port=6
  omega1 : Inport  Port=7
  psi1 : Inport  Port=8
  psi2 : Inport  Port=9
  psi3 : Inport  Port=10
  r1 : Inport  Port=11
  r2 : Inport  Port=12
  r3 : Inport  Port=13
  Add : Sum  Inputs=++++
  Subsystem3 : Subsystem
  Out1 : Outport
  wires:
  omega1/1 -> Add/1
  Subsystem3/2(Out2) -> Add/3
  phi12/1 -> Subsystem3/4(phiij2)
  Add/1 -> Out1/1
  phi11/1 -> Subsystem3/2(phiij1)
  Subsystem3/3(Out3) -> Add/4
  omega11/1 -> Subsystem3/1(omega11)
  Subsystem3/1(Out1) -> Add/2
  psi2/1 -> Subsystem3/8(psi2)
  omega12/1 -> Subsystem3/3(omega12)
  omega13/1 -> Subsystem3/5(omega13)
  phi13/1 -> Subsystem3/6(phiij3)
  psi1/1 -> Subsystem3/7(psi1)
  r3/1 -> Subsystem3/12(r3)
  r1/1 -> Subsystem3/10(r1)
  r2/1 -> Subsystem3/11(r2)
  psi3/1 -> Subsystem3/9(psi3)

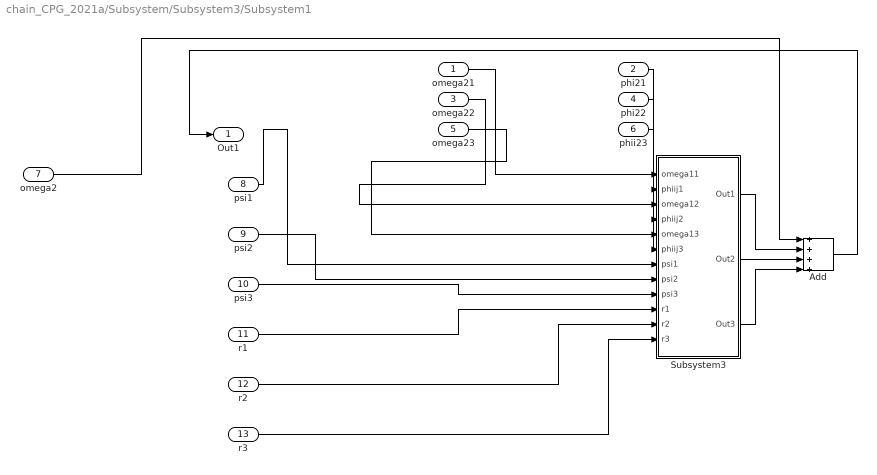
== system chain_CPG_2021a/Subsystem/Subsystem3/Subsystem1 ==
  omega21 : Inport
  phi21 : Inport  Port=2
  omega22 : Inport  Port=3
  phi22 : Inport  Port=4
  omega23 : Inport  Port=5
  phii23 : Inport  Port=6
  omega2 : Inport  Port=7
  psi1 : Inport  Port=8
  psi2 : Inport  Port=9
  psi3 : Inport  Port=10
  r1 : Inport  Port=11
  r2 : Inport  Port=12
  r3 : Inport  Port=13
  Add : Sum  Inputs=++++
  Subsystem3 : Subsystem
  Out1 : Outport
  wires:
  omega2/1 -> Add/1
  Subsystem3/2(Out2) -> Add/3
  phi22/1 -> Subsystem3/4(phiij2)
  Add/1 -> Out1/1
  phi21/1 -> Subsystem3/2(phiij1)
  Subsystem3/3(Out3) -> Add/4
  omega21/1 -> Subsystem3/1(omega11)
  Subsystem3/1(Out1) -> Add/2
  psi2/1 -> Subsystem3/8(psi2)
  omega22/1 -> Subsystem3/3(omega12)
  omega23/1 -> Subsystem3/5(omega13)
  phii23/1 -> Subsystem3/6(phiij3)
  psi1/1 -> Subsystem3/7(psi1)
  r3/1 -> Subsystem3/12(r3)
  r1/1 -> Subsystem3/10(r1)
  r2/1 -> Subsystem3/11(r2)
  psi3/1 -> Subsystem3/9(psi3)

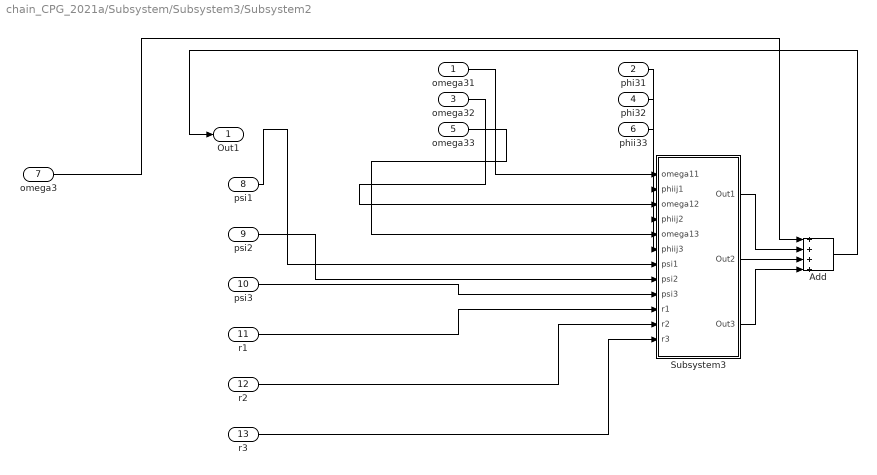
== system chain_CPG_2021a/Subsystem/Subsystem3/Subsystem2 ==
  omega31 : Inport
  phi31 : Inport  Port=2
  omega32 : Inport  Port=3
  phi32 : Inport  Port=4
  omega33 : Inport  Port=5
  phii33 : Inport  Port=6
  omega3 : Inport  Port=7
  psi1 : Inport  Port=8
  psi2 : Inport  Port=9
  psi3 : Inport  Port=10
  r1 : Inport  Port=11
  r2 : Inport  Port=12
  r3 : Inport  Port=13
  Add : Sum  Inputs=++++
  Subsystem3 : Subsystem
  Out1 : Outport
  wires:
  omega3/1 -> Add/1
  Subsystem3/2(Out2) -> Add/3
  phi32/1 -> Subsystem3/4(phiij2)
  Add/1 -> Out1/1
  phi31/1 -> Subsystem3/2(phiij1)
  Subsystem3/3(Out3) -> Add/4
  omega31/1 -> Subsystem3/1(omega11)
  Subsystem3/1(Out1) -> Add/2
  psi2/1 -> Subsystem3/8(psi2)
  omega32/1 -> Subsystem3/3(omega12)
  omega33/1 -> Subsystem3/5(omega13)
  phii33/1 -> Subsystem3/6(phiij3)
  psi1/1 -> Subsystem3/7(psi1)
  r3/1 -> Subsystem3/12(r3)
  r1/1 -> Subsystem3/10(r1)
  r2/1 -> Subsystem3/11(r2)
  psi3/1 -> Subsystem3/9(psi3)

== system chain_CPG_2021a/Subsystem/ddr/Subsystem3 ==
  ar : Inport
  Ri : Inport  Port=2
  ri : Inport  Port=3
  dri : Inport  Port=4
  Add : Sum  Inputs=+-
  Add1 : Sum  Inputs=+-
  Constant : Constant  Value=4
  Divide : Product  Inputs=*/
  Product : Product
  Product1 : Product
  ddri : Outport
  wires:
  Add1/1 -> Product/2
  dri/1 -> Add1/2
  Product1/1 -> Add1/1
  Divide/1 -> Product1/2
  Add/1 -> Product1/1
  Constant/1 -> Divide/2
  ri/1 -> Add/2
  Ri/1 -> Add/1
  Product/1 -> ddri/1
  ar/1 -> Divide/1, Product/1

== system chain_CPG_2021a/Subsystem/ddr/Subsystem4 ==
  ar : Inport
  Ri : Inport  Port=2
  ri : Inport  Port=3
  dri : Inport  Port=4
  Add : Sum  Inputs=+-
  Add1 : Sum  Inputs=+-
  Constant : Constant  Value=4
  Divide : Product  Inputs=*/
  Product : Product
  Product1 : Product
  ddri : Outport
  wires:
  Add1/1 -> Product/2
  dri/1 -> Add1/2
  Product1/1 -> Add1/1
  Divide/1 -> Product1/2
  Add/1 -> Product1/1
  Constant/1 -> Divide/2
  ri/1 -> Add/2
  Ri/1 -> Add/1
  Product/1 -> ddri/1
  ar/1 -> Divide/1, Product/1

== system chain_CPG_2021a/Subsystem/ddr/Subsystem5 ==
  ar : Inport
  Ri : Inport  Port=2
  ri : Inport  Port=3
  dri : Inport  Port=4
  Add : Sum  Inputs=+-
  Add1 : Sum  Inputs=+-
  Constant : Constant  Value=4
  Divide : Product  Inputs=*/
  Product : Product
  Product1 : Product
  ddri : Outport
  wires:
  Add1/1 -> Product/2
  dri/1 -> Add1/2
  Product1/1 -> Add1/1
  Divide/1 -> Product1/2
  Add/1 -> Product1/1
  Constant/1 -> Divide/2
  ri/1 -> Add/2
  Ri/1 -> Add/1
  Product/1 -> ddri/1
  ar/1 -> Divide/1, Product/1

== system chain_CPG_2021a/Subsystem/ddr1/Subsystem3 ==
  ar : Inport
  Ri : Inport  Port=2
  ri : Inport  Port=3
  dri : Inport  Port=4
  Add : Sum  Inputs=+-
  Add1 : Sum  Inputs=+-
  Constant : Constant  Value=4
  Divide : Product  Inputs=*/
  Product : Product
  Product1 : Product
  ddri : Outport
  wires:
  Add1/1 -> Product/2
  dri/1 -> Add1/2
  Product1/1 -> Add1/1
  Divide/1 -> Product1/2
  Add/1 -> Product1/1
  Constant/1 -> Divide/2
  ri/1 -> Add/2
  Ri/1 -> Add/1
  Product/1 -> ddri/1
  ar/1 -> Divide/1, Product/1

== system chain_CPG_2021a/Subsystem/ddr1/Subsystem4 ==
  ar : Inport
  Ri : Inport  Port=2
  ri : Inport  Port=3
  dri : Inport  Port=4
  Add : Sum  Inputs=+-
  Add1 : Sum  Inputs=+-
  Constant : Constant  Value=4
  Divide : Product  Inputs=*/
  Product : Product
  Product1 : Product
  ddri : Outport
  wires:
  Add1/1 -> Product/2
  dri/1 -> Add1/2
  Product1/1 -> Add1/1
  Divide/1 -> Product1/2
  Add/1 -> Product1/1
  Constant/1 -> Divide/2
  ri/1 -> Add/2
  Ri/1 -> Add/1
  Product/1 -> ddri/1
  ar/1 -> Divide/1, Product/1

== system chain_CPG_2021a/Subsystem/ddr1/Subsystem5 ==
  ar : Inport
  Ri : Inport  Port=2
  ri : Inport  Port=3
  dri : Inport  Port=4
  Add : Sum  Inputs=+-
  Add1 : Sum  Inputs=+-
  Constant : Constant  Value=4
  Divide : Product  Inputs=*/
  Product : Product
  Product1 : Product
  ddri : Outport
  wires:
  Add1/1 -> Product/2
  dri/1 -> Add1/2
  Product1/1 -> Add1/1
  Divide/1 -> Product1/2
  Add/1 -> Product1/1
  Constant/1 -> Divide/2
  ri/1 -> Add/2
  Ri/1 -> Add/1
  Product/1 -> ddri/1
  ar/1 -> Divide/1, Product/1

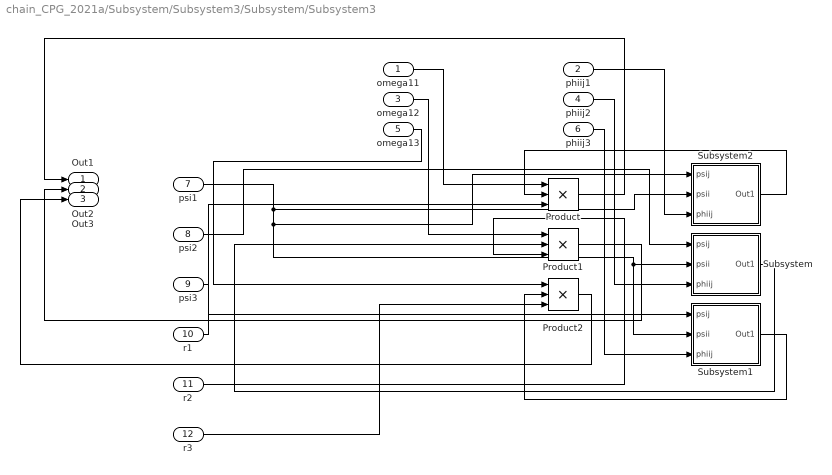
== system chain_CPG_2021a/Subsystem/Subsystem3/Subsystem/Subsystem3 ==
  omega11 : Inport
  phiij1 : Inport  Port=2
  omega12 : Inport  Port=3
  phiij2 : Inport  Port=4
  omega13 : Inport  Port=5
  phiij3 : Inport  Port=6
  psi1 : Inport  Port=7
  psi2 : Inport  Port=8
  psi3 : Inport  Port=9
  r1 : Inport  Port=10
  r2 : Inport  Port=11
  r3 : Inport  Port=12
  Product : Product  Inputs=3
  Product1 : Product  Inputs=3
  Product2 : Product  Inputs=3
  Subsystem : Subsystem
  Subsystem1 : Subsystem
  Subsystem2 : Subsystem
  Out1 : Outport
  Out2 : Outport  Port=2
  Out3 : Outport  Port=3
  wires:
  psi1/1 -> Subsystem2/1(psij), Subsystem1/2(psii), Subsystem/2(psii), Subsystem2/2(psii)
  phiij1/1 -> Subsystem2/3(phiij)
  psi3/1 -> Subsystem1/1(psij)
  r3/1 -> Product2/3
  Subsystem2/1(Out1) -> Product/2
  psi2/1 -> Subsystem/1(psij)
  phiij2/1 -> Subsystem/3(phiij)
  Subsystem/1(Out1) -> Product1/2
  Subsystem1/1(Out1) -> Product2/2
  omega11/1 -> Product/1
  r1/1 -> Product/3
  omega12/1 -> Product1/1
  r2/1 -> Product1/3
  Product/1 -> Out1/1
  phiij3/1 -> Subsystem1/3(phiij)
  Product2/1 -> Out3/1
  Product1/1 -> Out2/1
  omega13/1 -> Product2/1

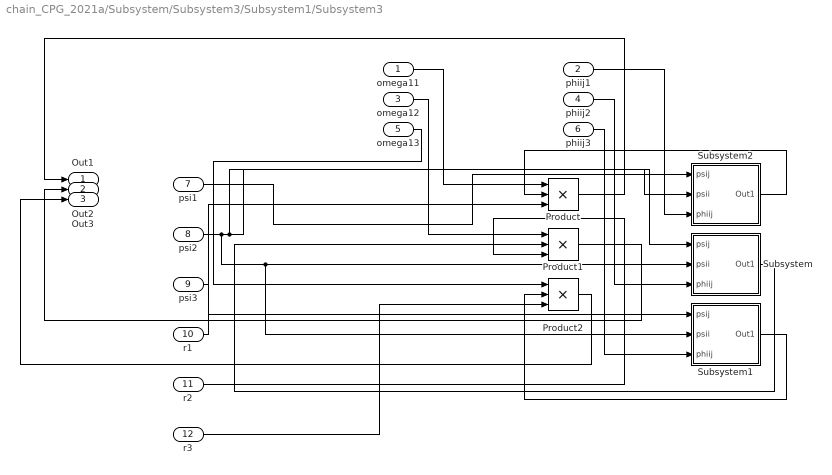
== system chain_CPG_2021a/Subsystem/Subsystem3/Subsystem1/Subsystem3 ==
  omega11 : Inport
  phiij1 : Inport  Port=2
  omega12 : Inport  Port=3
  phiij2 : Inport  Port=4
  omega13 : Inport  Port=5
  phiij3 : Inport  Port=6
  psi1 : Inport  Port=7
  psi2 : Inport  Port=8
  psi3 : Inport  Port=9
  r1 : Inport  Port=10
  r2 : Inport  Port=11
  r3 : Inport  Port=12
  Product : Product  Inputs=3
  Product1 : Product  Inputs=3
  Product2 : Product  Inputs=3
  Subsystem : Subsystem
  Subsystem1 : Subsystem
  Subsystem2 : Subsystem
  Out1 : Outport
  Out2 : Outport  Port=2
  Out3 : Outport  Port=3
  wires:
  psi1/1 -> Subsystem2/1(psij)
  phiij1/1 -> Subsystem2/3(phiij)
  psi3/1 -> Subsystem1/1(psij)
  r3/1 -> Product2/3
  Subsystem2/1(Out1) -> Product/2
  psi2/1 -> Subsystem1/2(psii), Subsystem/2(psii), Subsystem2/2(psii), Subsystem/1(psij)
  phiij2/1 -> Subsystem/3(phiij)
  Subsystem/1(Out1) -> Product1/2
  Subsystem1/1(Out1) -> Product2/2
  omega11/1 -> Product/1
  r1/1 -> Product/3
  omega12/1 -> Product1/1
  r2/1 -> Product1/3
  Product/1 -> Out1/1
  phiij3/1 -> Subsystem1/3(phiij)
  Product2/1 -> Out3/1
  Product1/1 -> Out2/1
  omega13/1 -> Product2/1

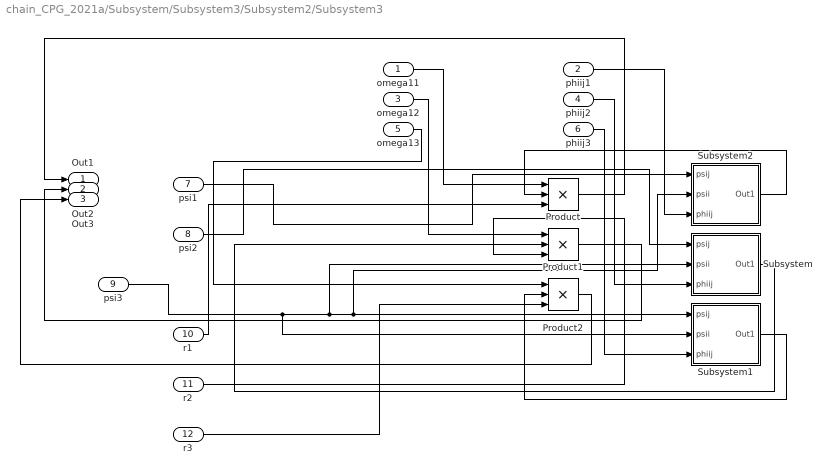
== system chain_CPG_2021a/Subsystem/Subsystem3/Subsystem2/Subsystem3 ==
  omega11 : Inport
  phiij1 : Inport  Port=2
  omega12 : Inport  Port=3
  phiij2 : Inport  Port=4
  omega13 : Inport  Port=5
  phiij3 : Inport  Port=6
  psi1 : Inport  Port=7
  psi2 : Inport  Port=8
  psi3 : Inport  Port=9
  r1 : Inport  Port=10
  r2 : Inport  Port=11
  r3 : Inport  Port=12
  Product : Product  Inputs=3
  Product1 : Product  Inputs=3
  Product2 : Product  Inputs=3
  Subsystem : Subsystem
  Subsystem1 : Subsystem
  Subsystem2 : Subsystem
  Out1 : Outport
  Out2 : Outport  Port=2
  Out3 : Outport  Port=3
  wires:
  psi1/1 -> Subsystem2/1(psij)
  phiij1/1 -> Subsystem2/3(phiij)
  r3/1 -> Product2/3
  Subsystem2/1(Out1) -> Product/2
  psi2/1 -> Subsystem/1(psij)
  phiij2/1 -> Subsystem/3(phiij)
  Subsystem/1(Out1) -> Product1/2
  Subsystem1/1(Out1) -> Product2/2
  omega11/1 -> Product/1
  r1/1 -> Product/3
  omega12/1 -> Product1/1
  r2/1 -> Product1/3
  Product/1 -> Out1/1
  phiij3/1 -> Subsystem1/3(phiij)
  Product2/1 -> Out3/1
  Product1/1 -> Out2/1
  omega13/1 -> Product2/1
  psi3/1 -> Subsystem1/2(psii), Subsystem/2(psii), Subsystem2/2(psii), Subsystem1/1(psij)

== system chain_CPG_2021a/Subsystem/Subsystem3/Subsystem/Subsystem3/Subsystem ==
  psij : Inport
  psii : Inport  Port=2
  phiij : Inport  Port=3
  Add1 : Sum  Inputs=+--
  Trigonometric Function1 : Trigonometry
  Out1 : Outport
  wires:
  psij/1 -> Add1/1
  phiij/1 -> Add1/3
  psii/1 -> Add1/2
  Add1/1 -> Trigonometric Function1/1
  Trigonometric Function1/1 -> Out1/1

== system chain_CPG_2021a/Subsystem/Subsystem3/Subsystem/Subsystem3/Subsystem1 ==
  psij : Inport
  psii : Inport  Port=2
  phiij : Inport  Port=3
  Add1 : Sum  Inputs=+--
  Trigonometric Function1 : Trigonometry
  Out1 : Outport
  wires:
  psij/1 -> Add1/1
  phiij/1 -> Add1/3
  psii/1 -> Add1/2
  Add1/1 -> Trigonometric Function1/1
  Trigonometric Function1/1 -> Out1/1

== system chain_CPG_2021a/Subsystem/Subsystem3/Subsystem/Subsystem3/Subsystem2 ==
  psij : Inport
  psii : Inport  Port=2
  phiij : Inport  Port=3
  Add1 : Sum  Inputs=+--
  Trigonometric Function1 : Trigonometry
  Out1 : Outport
  wires:
  psij/1 -> Add1/1
  phiij/1 -> Add1/3
  psii/1 -> Add1/2
  Add1/1 -> Trigonometric Function1/1
  Trigonometric Function1/1 -> Out1/1

== system chain_CPG_2021a/Subsystem/Subsystem3/Subsystem1/Subsystem3/Subsystem ==
  psij : Inport
  psii : Inport  Port=2
  phiij : Inport  Port=3
  Add1 : Sum  Inputs=+--
  Trigonometric Function1 : Trigonometry
  Out1 : Outport
  wires:
  psij/1 -> Add1/1
  phiij/1 -> Add1/3
  psii/1 -> Add1/2
  Add1/1 -> Trigonometric Function1/1
  Trigonometric Function1/1 -> Out1/1

== system chain_CPG_2021a/Subsystem/Subsystem3/Subsystem1/Subsystem3/Subsystem1 ==
  psij : Inport
  psii : Inport  Port=2
  phiij : Inport  Port=3
  Add1 : Sum  Inputs=+--
  Trigonometric Function1 : Trigonometry
  Out1 : Outport
  wires:
  psij/1 -> Add1/1
  phiij/1 -> Add1/3
  psii/1 -> Add1/2
  Add1/1 -> Trigonometric Function1/1
  Trigonometric Function1/1 -> Out1/1

== system chain_CPG_2021a/Subsystem/Subsystem3/Subsystem1/Subsystem3/Subsystem2 ==
  psij : Inport
  psii : Inport  Port=2
  phiij : Inport  Port=3
  Add1 : Sum  Inputs=+--
  Trigonometric Function1 : Trigonometry
  Out1 : Outport
  wires:
  psij/1 -> Add1/1
  phiij/1 -> Add1/3
  psii/1 -> Add1/2
  Add1/1 -> Trigonometric Function1/1
  Trigonometric Function1/1 -> Out1/1
